simulink model "unsteadyBEMTs"  (R2024b)
settings: Solver=VariableStepAuto  StartTime=0.0  StopTime=10.0  RelTol=1e-3
settings Model: Creator=thogan1  LastModifiedBy=thogan1

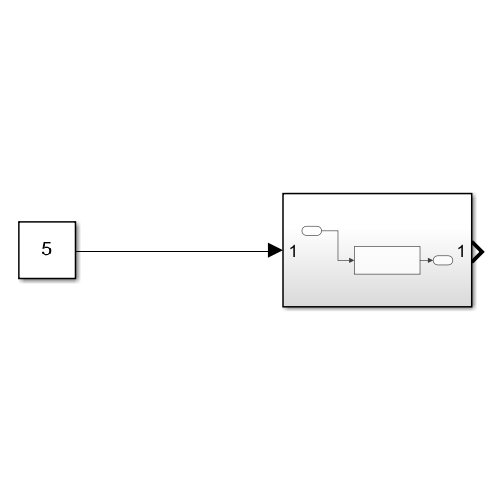
[thumbnail: Simulink's stored preview of the top-level diagram]
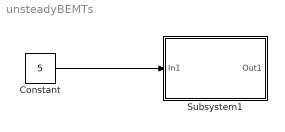
== system unsteadyBEMTs ==
  Constant : Constant  Value=5
  Subsystem1 : Subsystem
  wires:
  Constant/1 -> Subsystem1/1(In1)

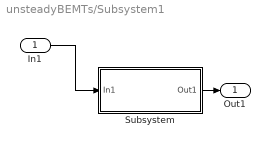
== system unsteadyBEMTs/Subsystem1 ==
  In1 : Inport
  Subsystem : Subsystem
  Out1 : Outport
  wires:
  Subsystem/1(Out1) -> Out1/1
  In1/1 -> Subsystem/1(In1)

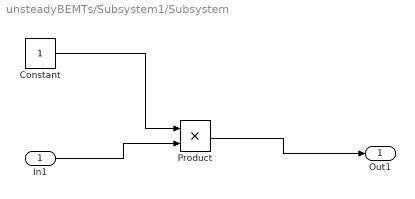
== system unsteadyBEMTs/Subsystem1/Subsystem ==
  In1 : Inport
  Constant : Constant
  Product : Product
  Out1 : Outport
  wires:
  Constant/1 -> Product/1
  In1/1 -> Product/2
  Product/1 -> Out1/1
